simulink model "park"  (R2021b)
settings: Solver=FixedStepDiscrete  StartTime=0.0  StopTime=10.0  FixedStep=1e-4  RelTol=1e-3
settings Model: DataDictionary=park.sldd  Creator=ssc  LastModifiedBy=ssc
settings OptimizationCC: DefaultParameterBehavior=Inlined  UseDivisionForNetSlopeComputation=on  GainParamInheritBuiltInType=on  UseFloatMulNetSlope=on  InlineInvariantSignals=on  PassReuseOutputArgsAs=Individual arguments  ZeroExternalMemoryAtStartup=off  ZeroInternalMemoryAtStartup=off  NoFixptDivByZeroProtection=on  EfficientFloat2IntCast=on  LifeSpan=1  OptimizeBlockOrder=speed  DifferentSizesBufferReuse=on  EfficientTunableParamExpr=on
settings DebuggingCC: ParameterTunabilityLossMsg=error
settings HardwareCC: ProdBitPerPointer=32  ProdBitPerSizeT=32  ProdBitPerPtrDiffT=32  ProdLargestAtomicInteger=Long  ProdLargestAtomicFloat=Double  ProdWordSize=32  ProdLongLongMode=on  ProdHWDeviceType=ARM Compatible->ARM Cortex-M
settings SFSimCC: MATLABDynamicMemAlloc=off
settings RTWCC: Description=Embedded Coder  SystemTargetFile=ert.tlc  TemplateMakefile=ert_default_tmf  GenerateReport=on  LaunchReport=on
settings CodeAppCC: ForceParamTrailComments=on  IgnoreCustomStorageClasses=off  OperatorAnnotations=on  SimulinkDataObjDesc=on  SFDataObjDesc=on  CustomSymbolStrGlobalVar=rt$N$M  CustomSymbolStrType=$N$M  CustomSymbolStrFcn=$N$M$F  CustomSymbolStrMacro=$N$M  InsertBlockDesc=on
settings ERTTargetCC: TargetLangStandard=C99 (ISO)  CodeReplacementLibrary=ARM Cortex-M  GenerateSampleERTMain=on  IncludeMdlTerminateFcn=off  CombineSignalStateStructs=on  SuppressErrorStatus=on  SupportAbsoluteTime=off  SupportNonFinite=off  SupportComplex=off  InlinedParameterPlacement=NonHierarchical  ERTCustomFileTemplate=example_file_process.tlc  ERTFilePackagingFormat=CompactWithDataFile

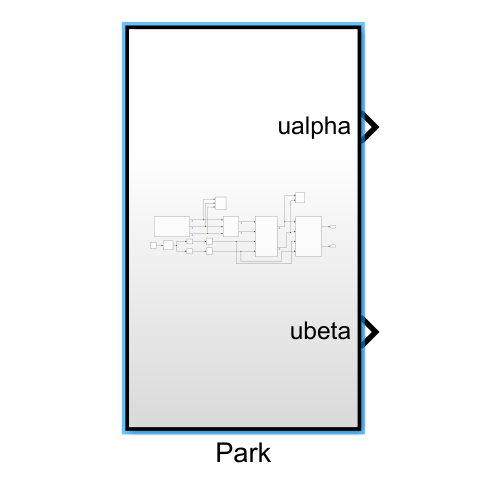
[thumbnail: Simulink's stored preview of the top-level diagram]
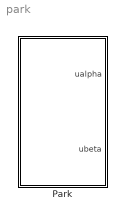
== system park ==
  Park : Subsystem  TreatAsAtomicUnit=on

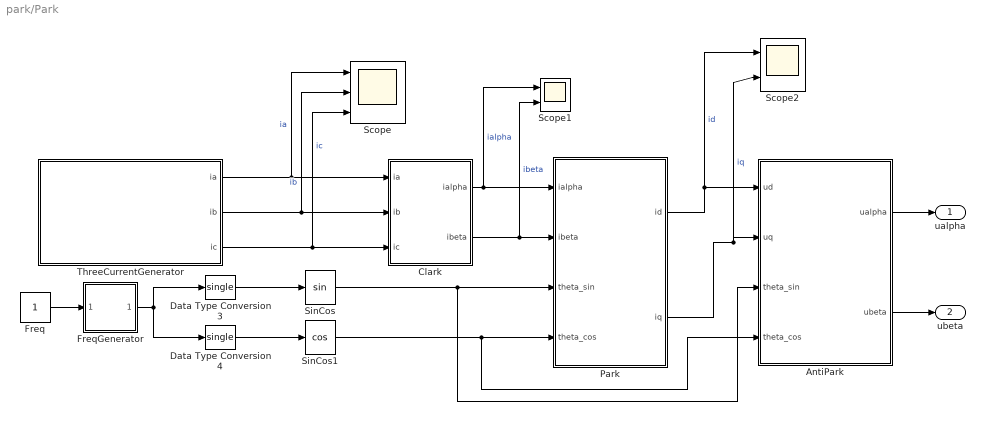
== system park/Park ==
  AntiPark : Subsystem
  Clark : Subsystem
  Data Type Conversion3 : DataTypeConversion  OutDataTypeStr=single
  Data Type Conversion4 : DataTypeConversion  OutDataTypeStr=single
  Freq : Constant  OutDataTypeStr=single
  FreqGenerator : Subsystem
  Park : Subsystem
  Scope : Scope  NumInputPorts=3
  Scope1 : Scope  NumInputPorts=2
  Scope2 : Scope  NumInputPorts=2
  SinCos : Trigonometry  ApproximationMethod=Lookup
  SinCos1 : Trigonometry  Operator=cos  ApproximationMethod=Lookup
  ThreeCurrentGenerator : Subsystem
  ualpha : Outport
  ubeta : Outport  Port=2
  wires:
  ThreeCurrentGenerator/1(ia) -> Clark/1(ia), Scope/1  "ia"
  ThreeCurrentGenerator/3(ic) -> Clark/3(ic), Scope/3  "ic"
  ThreeCurrentGenerator/2(ib) -> Clark/2(ib), Scope/2  "ib"
  Data Type Conversion3/1 -> SinCos/1
  FreqGenerator/1(Theta) -> Data Type Conversion4/1, Data Type Conversion3/1
  Freq/1 -> FreqGenerator/1(Freq)
  Data Type Conversion4/1 -> SinCos1/1
  Clark/1(ialpha) -> Scope1/1, Park/1(ialpha)  "ialpha"
  Clark/2(ibeta) -> Scope1/2, Park/2(ibeta)  "ibeta"
  SinCos/1 -> AntiPark/3(theta_sin), Park/3(theta_sin)
  SinCos1/1 -> AntiPark/4(theta_cos), Park/4(theta_cos)
  Park/1(id) -> Scope2/1, AntiPark/1(ud)  "id"
  Park/2(iq) -> Scope2/2, AntiPark/2(uq)  "iq"
  AntiPark/2(ubeta) -> ubeta/1
  AntiPark/1(ualpha) -> ualpha/1

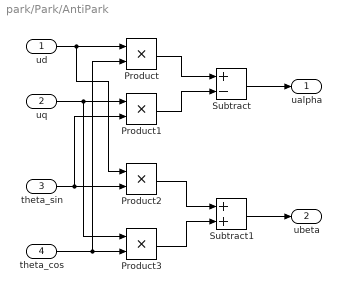
== system park/Park/AntiPark ==
  ud : Inport
  uq : Inport  Port=2
  theta_sin : Inport  Port=3
  theta_cos : Inport  Port=4
  Product{,1..3} (4 alike) : Product
  Subtract : Sum  Inputs=+-
  Subtract1 : Sum
  ualpha : Outport
  ubeta : Outport  Port=2
  wires:
  Product3/1 -> Subtract1/2
  theta_cos/1 -> Product/2, Product3/2
  Product1/1 -> Subtract/2
  ud/1 -> Product2/1, Product/1
  Product/1 -> Subtract/1
  theta_sin/1 -> Product1/2, Product2/2
  uq/1 -> Product3/1, Product1/1
  Subtract1/1 -> ubeta/1
  Product2/1 -> Subtract1/1
  Subtract/1 -> ualpha/1

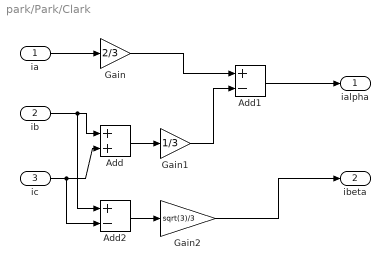
== system park/Park/Clark ==
  ia : Inport  OutDataTypeStr=single
  ib : Inport  Port=2  OutDataTypeStr=single
  ic : Inport  Port=3  OutDataTypeStr=single
  Add : Sum  AccumDataTypeStr=single  OutDataTypeStr=single
  Add1 : Sum  Inputs=+-  AccumDataTypeStr=single  OutDataTypeStr=single
  Add2 : Sum  Inputs=+-  AccumDataTypeStr=single  OutDataTypeStr=single
  Gain : Gain  Gain=2/3  ParamDataTypeStr=single
  Gain1 : Gain  Gain=1/3  ParamDataTypeStr=single
  Gain2 : Gain  Gain=sqrt(3)/3  ParamDataTypeStr=single
  ialpha : Outport  OutDataTypeStr=single
  ibeta : Outport  Port=2  OutDataTypeStr=single
  wires:
  ic/1 -> Add2/2, Add/2
  Gain1/1 -> Add1/2
  Gain/1 -> Add1/1
  Add/1 -> Gain1/1
  Add1/1 -> ialpha/1
  ib/1 -> Add2/1, Add/1
  ia/1 -> Gain/1
  Add2/1 -> Gain2/1
  Gain2/1 -> ibeta/1

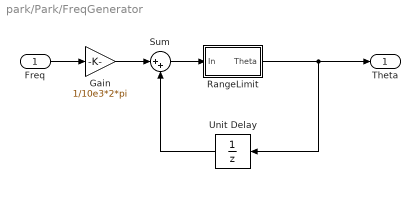
== system park/Park/FreqGenerator ==
  Freq : Inport
  Gain : Gain  Gain=1/10e3*2*pi  OutDataTypeStr=single
  RangeLimit : Subsystem
  Sum : Sum  Inputs=|++  OutDataTypeStr=Inherit: Same as first input
  Unit Delay : UnitDelay  SampleTime=-1  HasFrameUpgradeWarning=on
  Theta : Outport
  wires:
  Freq/1 -> Gain/1
  RangeLimit/1(Theta) -> Theta/1, Unit Delay/1
  Gain/1 -> Sum/1
  Sum/1 -> RangeLimit/1(In)
  Unit Delay/1 -> Sum/2

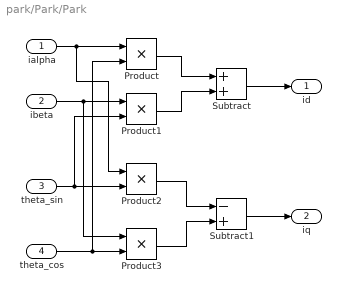
== system park/Park/Park ==
  ialpha : Inport
  ibeta : Inport  Port=2
  theta_sin : Inport  Port=3
  theta_cos : Inport  Port=4
  Product{,1..3} (4 alike) : Product
  Subtract : Sum
  Subtract1 : Sum  Inputs=-+
  id : Outport
  iq : Outport  Port=2
  wires:
  ialpha/1 -> Product2/1, Product/1
  theta_cos/1 -> Product/2, Product3/2
  ibeta/1 -> Product3/1, Product1/1
  theta_sin/1 -> Product1/2, Product2/2
  Product/1 -> Subtract/1
  Product1/1 -> Subtract/2
  Subtract/1 -> id/1
  Product2/1 -> Subtract1/1
  Product3/1 -> Subtract1/2
  Subtract1/1 -> iq/1

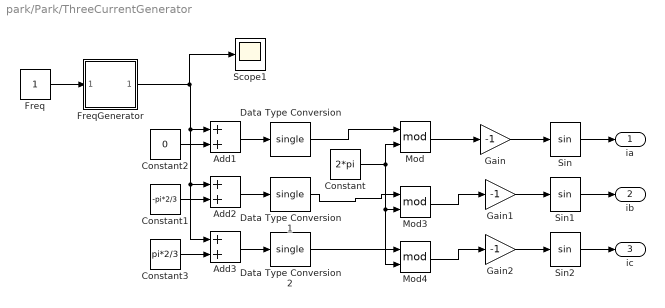
== system park/Park/ThreeCurrentGenerator ==
  Add1 : Sum  AccumDataTypeStr=single  OutDataTypeStr=single
  Add2 : Sum  AccumDataTypeStr=single  OutDataTypeStr=single
  Add3 : Sum  AccumDataTypeStr=single  OutDataTypeStr=single
  Constant : Constant  Value=2*pi  OutDataTypeStr=single
  Constant1 : Constant  Value=-pi*2/3  OutDataTypeStr=single
  Constant2 : Constant  Value=0  OutDataTypeStr=single
  Constant3 : Constant  Value=pi*2/3  OutDataTypeStr=single
  Data Type Conversion : DataTypeConversion  OutDataTypeStr=single
  Data Type Conversion1 : DataTypeConversion  OutDataTypeStr=single
  Data Type Conversion2 : DataTypeConversion  OutDataTypeStr=single
  Freq : Constant  OutDataTypeStr=single
  FreqGenerator : Subsystem
  Gain : Gain  Gain=-1
  Gain1 : Gain  Gain=-1
  Gain2 : Gain  Gain=-1
  Mod : Math  Operator=mod  SaturateOnIntegerOverflow=on
  Mod3 : Math  Operator=mod  SaturateOnIntegerOverflow=on
  Mod4 : Math  Operator=mod  SaturateOnIntegerOverflow=on
  Scope1 : Scope
  Sin : Trigonometry  ApproximationMethod=Lookup
  Sin1 : Trigonometry  ApproximationMethod=Lookup
  Sin2 : Trigonometry  ApproximationMethod=Lookup
  ia : Outport
  ib : Outport  Port=2
  ic : Outport  Port=3
  wires:
  Data Type Conversion1/1 -> Mod3/1
  Data Type Conversion2/1 -> Mod4/1
  Add1/1 -> Data Type Conversion/1
  Add2/1 -> Data Type Conversion1/1
  Add3/1 -> Data Type Conversion2/1
  Mod4/1 -> Gain2/1
  FreqGenerator/1(Theta) -> Scope1/1, Add3/1, Add2/1, Add1/1
  Data Type Conversion/1 -> Mod/1
  Gain2/1 -> Sin2/1
  Mod3/1 -> Gain1/1
  Mod/1 -> Gain/1
  Freq/1 -> FreqGenerator/1(Freq)
  Constant/1 -> Mod4/2, Mod3/2, Mod/2
  Constant2/1 -> Add1/2
  Gain/1 -> Sin/1
  Sin/1 -> ia/1
  Constant1/1 -> Add2/2
  Sin1/1 -> ib/1
  Sin2/1 -> ic/1
  Constant3/1 -> Add3/2
  Gain1/1 -> Sin1/1

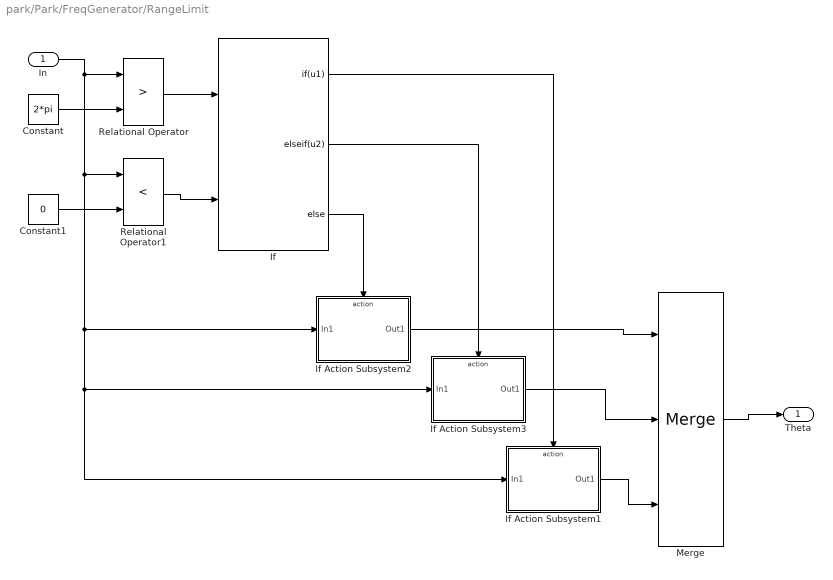
== system park/Park/FreqGenerator/RangeLimit ==
  In : Inport
  Constant : Constant  Value=2*pi  OutDataTypeStr=single  SampleTime=-1
  Constant1 : Constant  Value=0  OutDataTypeStr=single  SampleTime=-1
  If : If  NumInputs=2  IfExpression=u1  ElseIfExpressions=u2
  If Action Subsystem1 : Subsystem  TreatAsAtomicUnit=on
  If Action Subsystem2 : Subsystem  TreatAsAtomicUnit=on
  If Action Subsystem3 : Subsystem  TreatAsAtomicUnit=on
  Merge : Merge  Inputs=3
  Relational Operator : RelationalOperator  Operator=>  OutDataTypeStr=boolean  RndMeth=Simplest
  Relational Operator1 : RelationalOperator  Operator=<  OutDataTypeStr=boolean  RndMeth=Simplest
  Theta : Outport
  wires:
  Relational Operator/1 -> If/1
  Constant/1 -> Relational Operator/2
  In/1 -> Relational Operator1/1, If Action Subsystem2/1(In1), If Action Subsystem3/1(In1), If Action Subsystem1/1(In1), Relational Operator/1
  Merge/1 -> Theta/1
  If/3 -> If Action Subsystem2/Action
  If/1 -> If Action Subsystem1/Action
  If Action Subsystem2/1(Out1) -> Merge/1
  Constant1/1 -> Relational Operator1/2
  Relational Operator1/1 -> If/2
  If/2 -> If Action Subsystem3/Action
  If Action Subsystem1/1(Out1) -> Merge/3
  If Action Subsystem3/1(Out1) -> Merge/2

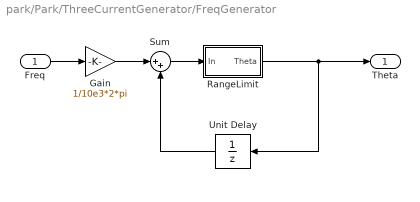
== system park/Park/ThreeCurrentGenerator/FreqGenerator ==
  Freq : Inport
  Gain : Gain  Gain=1/10e3*2*pi  OutDataTypeStr=single
  RangeLimit : Subsystem
  Sum : Sum  Inputs=|++  OutDataTypeStr=Inherit: Same as first input
  Unit Delay : UnitDelay  SampleTime=-1  HasFrameUpgradeWarning=on
  Theta : Outport
  wires:
  Freq/1 -> Gain/1
  RangeLimit/1(Theta) -> Theta/1, Unit Delay/1
  Gain/1 -> Sum/1
  Sum/1 -> RangeLimit/1(In)
  Unit Delay/1 -> Sum/2

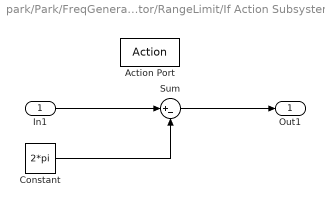
== system park/Park/FreqGenerator/RangeLimit/If Action Subsystem1 ==
  In1 : Inport
  Action Port : ActionPort  ActionPortLabel=if(u1)
  Constant : Constant  Value=2*pi  OutDataTypeStr=single  SampleTime=-1
  Sum : Sum  Inputs=|+-
  Out1 : Outport
  wires:
  In1/1 -> Sum/1
  Constant/1 -> Sum/2
  Sum/1 -> Out1/1

== system park/Park/FreqGenerator/RangeLimit/If Action Subsystem2 ==
  In1 : Inport
  Action Port : ActionPort  ActionPortLabel=else
  Out1 : Outport
  wires:
  In1/1 -> Out1/1

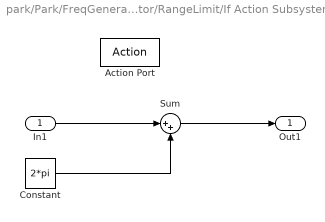
== system park/Park/FreqGenerator/RangeLimit/If Action Subsystem3 ==
  In1 : Inport
  Action Port : ActionPort  ActionPortLabel=elseif(u2)
  Constant : Constant  Value=2*pi  OutDataTypeStr=single  SampleTime=-1
  Sum : Sum  Inputs=|++
  Out1 : Outport
  wires:
  Constant/1 -> Sum/2
  In1/1 -> Sum/1
  Sum/1 -> Out1/1

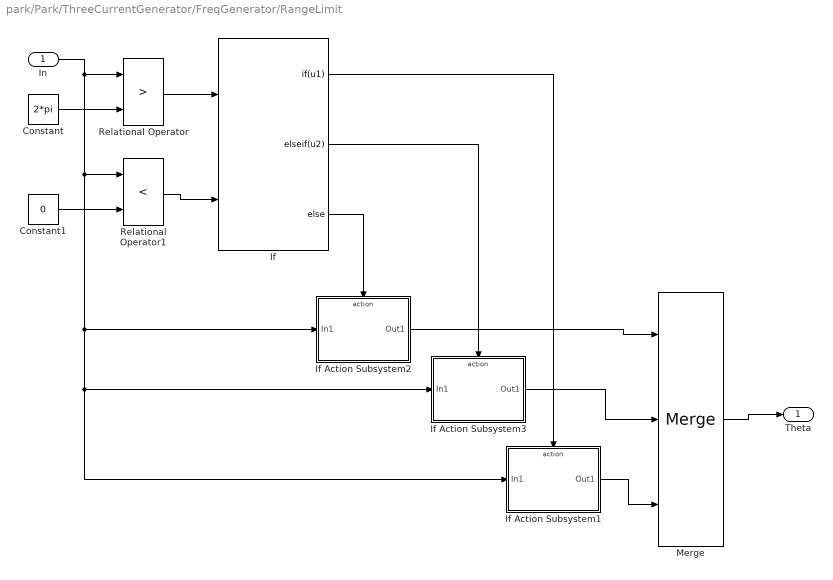
== system park/Park/ThreeCurrentGenerator/FreqGenerator/RangeLimit ==
  In : Inport
  Constant : Constant  Value=2*pi  OutDataTypeStr=single  SampleTime=-1
  Constant1 : Constant  Value=0  OutDataTypeStr=single  SampleTime=-1
  If : If  NumInputs=2  IfExpression=u1  ElseIfExpressions=u2
  If Action Subsystem1 : Subsystem  TreatAsAtomicUnit=on
  If Action Subsystem2 : Subsystem  TreatAsAtomicUnit=on
  If Action Subsystem3 : Subsystem  TreatAsAtomicUnit=on
  Merge : Merge  Inputs=3
  Relational Operator : RelationalOperator  Operator=>  OutDataTypeStr=boolean  RndMeth=Simplest
  Relational Operator1 : RelationalOperator  Operator=<  OutDataTypeStr=boolean  RndMeth=Simplest
  Theta : Outport
  wires:
  Relational Operator/1 -> If/1
  Constant/1 -> Relational Operator/2
  In/1 -> Relational Operator1/1, If Action Subsystem2/1(In1), If Action Subsystem3/1(In1), If Action Subsystem1/1(In1), Relational Operator/1
  Merge/1 -> Theta/1
  If/3 -> If Action Subsystem2/Action
  If/1 -> If Action Subsystem1/Action
  If Action Subsystem2/1(Out1) -> Merge/1
  Constant1/1 -> Relational Operator1/2
  Relational Operator1/1 -> If/2
  If/2 -> If Action Subsystem3/Action
  If Action Subsystem1/1(Out1) -> Merge/3
  If Action Subsystem3/1(Out1) -> Merge/2

== system park/Park/ThreeCurrentGenerator/FreqGenerator/RangeLimit/If Action Subsystem1 ==
  In1 : Inport
  Action Port : ActionPort  ActionPortLabel=if(u1)
  Constant : Constant  Value=2*pi  OutDataTypeStr=single  SampleTime=-1
  Sum : Sum  Inputs=|+-
  Out1 : Outport
  wires:
  In1/1 -> Sum/1
  Constant/1 -> Sum/2
  Sum/1 -> Out1/1

== system park/Park/ThreeCurrentGenerator/FreqGenerator/RangeLimit/If Action Subsystem2 ==
  In1 : Inport
  Action Port : ActionPort  ActionPortLabel=else
  Out1 : Outport
  wires:
  In1/1 -> Out1/1

== system park/Park/ThreeCurrentGenerator/FreqGenerator/RangeLimit/If Action Subsystem3 ==
  In1 : Inport
  Action Port : ActionPort  ActionPortLabel=elseif(u2)
  Constant : Constant  Value=2*pi  OutDataTypeStr=single  SampleTime=-1
  Sum : Sum  Inputs=|++
  Out1 : Outport
  wires:
  Constant/1 -> Sum/2
  In1/1 -> Sum/1
  Sum/1 -> Out1/1
